simulink model "Kinect_Block_modified"  (R2012b)
settings: Solver=ode45  StartTime=0.0  StopTime=inf  RelTol=1e-3
undefined symbols (not defined in the file or in its folder): gray
libraries: nid_lib x2, visionsinks x1, utility x1
settings Model: Creator=Eka  LastModifiedBy=Eka

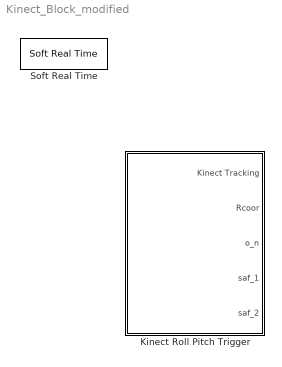
== system Kinect_Block_modified ==
  Kinect Roll Pitch Trigger : Subsystem
  Soft Real Time : utility/Soft Real Time  x=0.8

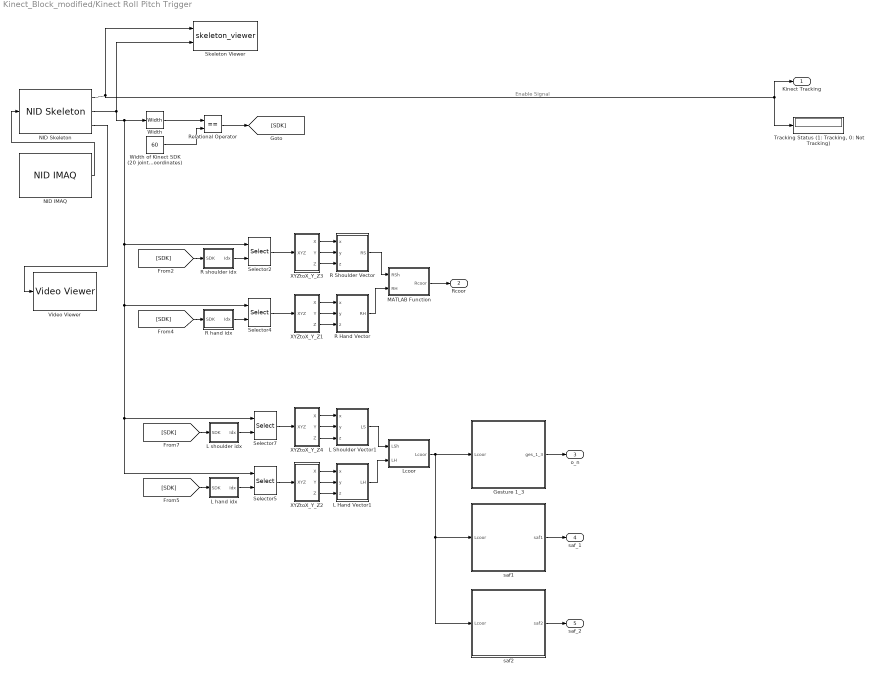
== system Kinect_Block_modified/Kinect Roll Pitch Trigger ==
  note: Enable Signal
  Gesture 1_3 : MATLAB Function  TreatAsAtomicUnit=on
  L Hand Vector1 : MATLAB Function  TreatAsAtomicUnit=on
  L Shoulder Vector1 : MATLAB Function  TreatAsAtomicUnit=on
  L hand idx : Subsystem
  L shoulder idx : Subsystem
  Lcoor : MATLAB Function  TreatAsAtomicUnit=on
  MATLAB Function : MATLAB Function  TreatAsAtomicUnit=on
  NID IMAQ : nid_lib/NID IMAQ  imaq_depth=off  imaq_motion=off  imaq_image=off  view_point=off  imaq_skeleton=on  imaq_ir=off  mirror_image=off  imaq_sample_time=1/25  res_fps=VGA (640x480): 30 FPS  needPsiPose=off  angle_input=off  angle=0  angle_read=off  near_mode=on  seated_mode=on  skeleton_smooth=[1.0 0.5 0.5 0.05 0.04]  infer_skeleton=on
  NID Skeleton : nid_lib/NID Skeleton  num_of_skeleton_tracking=1  conv_XYZ_RW=on  viewer=on
  R Hand Vector : MATLAB Function  TreatAsAtomicUnit=on
  R Shoulder Vector : MATLAB Function  TreatAsAtomicUnit=on
  R hand idx : Subsystem
  R shoulder idx : Subsystem
  Relational Operator : RelationalOperator  Operator===  OutDataTypeStr=boolean
  Selector{2,4..5,7} (4 alike) : Selector  NumberOfDimensions=3  InputPortWidth=3  IndexOptions=Select all,Index vector (port),Select all  Indices=[1 3],1,1  OutputSizes=1,1,1
  Skeleton Viewer : M-S-Function  FunctionName=skeleton_viewer
      mask Display:
      | disp('Skeleton\nViewer')
      | 
      | port_label('input', 1, 'Tracking')
      | port_label('input', 2, 'Skeleton')
  "Tracking Status (1: Tracking, 0: Not Tracking)" : Display
  Video Viewer : visionsinks/Video Viewer  inputType=Obsolete7b  imagePorts=One multidimensional signal  useColorMap=off  colormapValue=gray(256)  specRange=off  minInputVal=0  maxInputVal=255  FigPos=[578 777 794 668]  AxisZoom=on  trueSizedOnce=off  OpenAtMdlStart=on  DefaultConfigurationName=vipscopes.VideoViewerScopeCfg
  Width : Width
  Width of Kinect SDK (20 joints x 3 coordinates) : Constant  Value=60
  XYZtoX_Y_Z1 : Subsystem
  XYZtoX_Y_Z2 : Subsystem
  XYZtoX_Y_Z3 : Subsystem
  XYZtoX_Y_Z4 : Subsystem
  saf1 : MATLAB Function  TreatAsAtomicUnit=on
  saf2 : MATLAB Function  TreatAsAtomicUnit=on
  Kinect Tracking : Outport
  Rcoor : Outport  Port=2
  o_n : Outport  Port=3
  saf_1 : Outport  Port=4
  saf_2 : Outport  Port=5
  wires:
  [SDK] -> R hand idx/1(SDK)
  R hand idx/1(Idx) -> Selector4/2
  [SDK] -> R shoulder idx/1(SDK)
  R shoulder idx/1(Idx) -> Selector2/2
  NID Skeleton/1 -> "Tracking Status (1: Tracking, 0: Not Tracking)"/1, Kinect Tracking/1, Skeleton Viewer/1
  Relational Operator/1 -> [SDK]
  Width of Kinect SDK (20 joints x 3 coordinates)/1 -> Relational Operator/2
  Width/1 -> Relational Operator/1
  NID IMAQ/1 -> NID Skeleton/1
  [SDK] -> L hand idx/1(SDK)
  [SDK] -> L shoulder idx/1(SDK)
  L hand idx/1(Idx) -> Selector5/2
  L shoulder idx/1(Idx) -> Selector7/2
  NID Skeleton/3 -> Video Viewer/1
  NID Skeleton/2 -> Selector5/1, Selector7/1, Selector4/1, Selector2/1, Width/1, Skeleton Viewer/2
  MATLAB Function/1(Rcoor) -> Rcoor/1
  Selector2/1 -> XYZtoX_Y_Z3/1(XYZ)
  Selector4/1 -> XYZtoX_Y_Z1/1(XYZ)
  XYZtoX_Y_Z1/1(X) -> R Hand Vector/1(x)
  XYZtoX_Y_Z1/2(Y) -> R Hand Vector/2(y)
  XYZtoX_Y_Z1/3(Z) -> R Hand Vector/3(z)
  XYZtoX_Y_Z3/3(Z) -> R Shoulder Vector/3(z)
  XYZtoX_Y_Z3/2(Y) -> R Shoulder Vector/2(y)
  XYZtoX_Y_Z3/1(X) -> R Shoulder Vector/1(x)
  R Shoulder Vector/1(RS) -> MATLAB Function/1(RSh)
  R Hand Vector/1(RH) -> MATLAB Function/2(RH)
  XYZtoX_Y_Z2/1(X) -> L Hand Vector1/1(x)
  XYZtoX_Y_Z2/2(Y) -> L Hand Vector1/2(y)
  XYZtoX_Y_Z2/3(Z) -> L Hand Vector1/3(z)
  XYZtoX_Y_Z4/3(Z) -> L Shoulder Vector1/3(z)
  XYZtoX_Y_Z4/2(Y) -> L Shoulder Vector1/2(y)
  XYZtoX_Y_Z4/1(X) -> L Shoulder Vector1/1(x)
  Selector7/1 -> XYZtoX_Y_Z4/1(XYZ)
  Selector5/1 -> XYZtoX_Y_Z2/1(XYZ)
  L Shoulder Vector1/1(LS) -> Lcoor/1(LSh)
  L Hand Vector1/1(LH) -> Lcoor/2(LH)
  Lcoor/1(Lcoor) -> Gesture 1_3/1(Lcoor), saf2/1(Lcoor), saf1/1(Lcoor)
  saf1/1(saf1) -> saf_1/1
  saf2/1(saf2) -> saf_2/1
  Gesture 1_3/1(ges_1_3) -> o_n/1

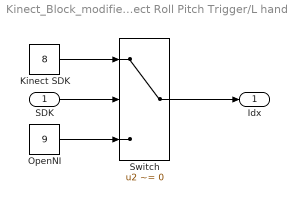
== system Kinect_Block_modified/Kinect Roll Pitch Trigger/L hand idx ==
  SDK : Inport
  Kinect SDK : Constant  Value=8
  OpenNI : Constant  Value=9
  Switch : Switch  Criteria=u2 ~= 0
  Idx : Outport
  wires:
  Kinect SDK/1 -> Switch/1
  OpenNI/1 -> Switch/3
  SDK/1 -> Switch/2
  Switch/1 -> Idx/1

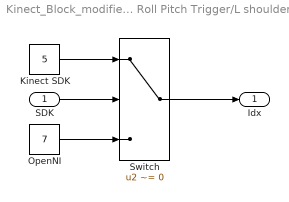
== system Kinect_Block_modified/Kinect Roll Pitch Trigger/L shoulder idx ==
  SDK : Inport
  Kinect SDK : Constant  Value=5
  OpenNI : Constant  Value=7
  Switch : Switch  Criteria=u2 ~= 0
  Idx : Outport
  wires:
  Kinect SDK/1 -> Switch/1
  OpenNI/1 -> Switch/3
  SDK/1 -> Switch/2
  Switch/1 -> Idx/1

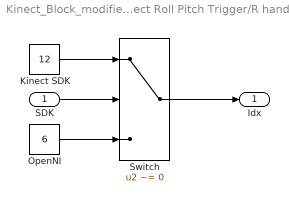
== system Kinect_Block_modified/Kinect Roll Pitch Trigger/R hand idx ==
  SDK : Inport
  Kinect SDK : Constant  Value=12
  OpenNI : Constant  Value=6
  Switch : Switch  Criteria=u2 ~= 0
  Idx : Outport
  wires:
  Switch/1 -> Idx/1
  SDK/1 -> Switch/2
  OpenNI/1 -> Switch/3
  Kinect SDK/1 -> Switch/1

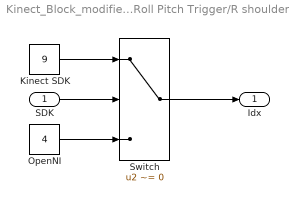
== system Kinect_Block_modified/Kinect Roll Pitch Trigger/R shoulder idx ==
  SDK : Inport
  Kinect SDK : Constant  Value=9
  OpenNI : Constant  Value=4
  Switch : Switch  Criteria=u2 ~= 0
  Idx : Outport
  wires:
  Switch/1 -> Idx/1
  SDK/1 -> Switch/2
  OpenNI/1 -> Switch/3
  Kinect SDK/1 -> Switch/1

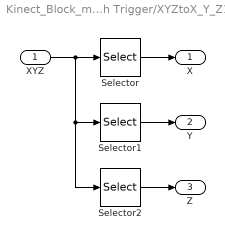
== system Kinect_Block_modified/Kinect Roll Pitch Trigger/XYZtoX_Y_Z1 ==
  XYZ : Inport
  Selector : Selector  NumberOfDimensions=3  InputPortWidth=3  IndexOptions=Index vector (dialog),Index vector (dialog),Index vector (dialog)  Indices=1,1,1  OutputSizes=1,1,1
  Selector1 : Selector  NumberOfDimensions=3  InputPortWidth=3  IndexOptions=Index vector (dialog),Index vector (dialog),Index vector (dialog)  Indices=1,1,2  OutputSizes=1,1,1
  Selector2 : Selector  NumberOfDimensions=3  InputPortWidth=3  IndexOptions=Index vector (dialog),Index vector (dialog),Index vector (dialog)  Indices=1,1,3  OutputSizes=1,1,1
  X : Outport
  Y : Outport  Port=2
  Z : Outport  Port=3
  wires:
  Selector2/1 -> Z/1
  Selector1/1 -> Y/1
  Selector/1 -> X/1
  XYZ/1 -> Selector2/1, Selector1/1, Selector/1

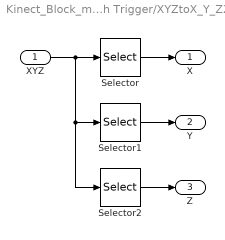
== system Kinect_Block_modified/Kinect Roll Pitch Trigger/XYZtoX_Y_Z2 ==
  XYZ : Inport
  Selector : Selector  NumberOfDimensions=3  InputPortWidth=3  IndexOptions=Index vector (dialog),Index vector (dialog),Index vector (dialog)  Indices=1,1,1  OutputSizes=1,1,1
  Selector1 : Selector  NumberOfDimensions=3  InputPortWidth=3  IndexOptions=Index vector (dialog),Index vector (dialog),Index vector (dialog)  Indices=1,1,2  OutputSizes=1,1,1
  Selector2 : Selector  NumberOfDimensions=3  InputPortWidth=3  IndexOptions=Index vector (dialog),Index vector (dialog),Index vector (dialog)  Indices=1,1,3  OutputSizes=1,1,1
  X : Outport
  Y : Outport  Port=2
  Z : Outport  Port=3
  wires:
  XYZ/1 -> Selector/1, Selector1/1, Selector2/1
  Selector/1 -> X/1
  Selector1/1 -> Y/1
  Selector2/1 -> Z/1

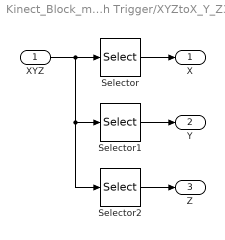
== system Kinect_Block_modified/Kinect Roll Pitch Trigger/XYZtoX_Y_Z3 ==
  XYZ : Inport
  Selector : Selector  NumberOfDimensions=3  InputPortWidth=3  IndexOptions=Index vector (dialog),Index vector (dialog),Index vector (dialog)  Indices=1,1,1  OutputSizes=1,1,1
  Selector1 : Selector  NumberOfDimensions=3  InputPortWidth=3  IndexOptions=Index vector (dialog),Index vector (dialog),Index vector (dialog)  Indices=1,1,2  OutputSizes=1,1,1
  Selector2 : Selector  NumberOfDimensions=3  InputPortWidth=3  IndexOptions=Index vector (dialog),Index vector (dialog),Index vector (dialog)  Indices=1,1,3  OutputSizes=1,1,1
  X : Outport
  Y : Outport  Port=2
  Z : Outport  Port=3
  wires:
  XYZ/1 -> Selector/1, Selector1/1, Selector2/1
  Selector/1 -> X/1
  Selector1/1 -> Y/1
  Selector2/1 -> Z/1

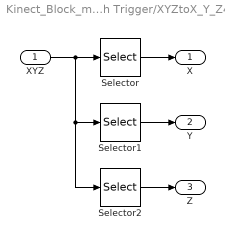
== system Kinect_Block_modified/Kinect Roll Pitch Trigger/XYZtoX_Y_Z4 ==
  XYZ : Inport
  Selector : Selector  NumberOfDimensions=3  InputPortWidth=3  IndexOptions=Index vector (dialog),Index vector (dialog),Index vector (dialog)  Indices=1,1,1  OutputSizes=1,1,1
  Selector1 : Selector  NumberOfDimensions=3  InputPortWidth=3  IndexOptions=Index vector (dialog),Index vector (dialog),Index vector (dialog)  Indices=1,1,2  OutputSizes=1,1,1
  Selector2 : Selector  NumberOfDimensions=3  InputPortWidth=3  IndexOptions=Index vector (dialog),Index vector (dialog),Index vector (dialog)  Indices=1,1,3  OutputSizes=1,1,1
  X : Outport
  Y : Outport  Port=2
  Z : Outport  Port=3
  wires:
  Selector2/1 -> Z/1
  Selector1/1 -> Y/1
  Selector/1 -> X/1
  XYZ/1 -> Selector2/1, Selector1/1, Selector/1

== matlab function Kinect_Block_modified/Kinect Roll Pitch Trigger/L Hand Vector1 ==
  data: x input; y input; z input; LH output
function LH = fcn(x,y,z)
LH = [x,y,z];

== matlab function Kinect_Block_modified/Kinect Roll Pitch Trigger/Lcoor ==
  data: LSh input; LH input; Lcoor output
function Lcoor = fcn(LSh, LH)
%#codegen

Lcoor = (LH - LSh)*10;

== matlab function Kinect_Block_modified/Kinect Roll Pitch Trigger/MATLAB Function ==
  data: RSh input; RH input; Rcoor output
function Rcoor = fcn(RSh, RH)

x_axis = (RH(1) - RSh(1))*(-5);
y_axis = ((RH(3) - RSh(3))+4)*4/3;
z_axis = (((RH(2) - RSh(2))+1)*1.8/7)-1.5;
Rcoor = [x_axis, y_axis, z_axis];

== matlab function Kinect_Block_modified/Kinect Roll Pitch Trigger/L Shoulder Vector1 ==
  data: x input; y input; z input; LS output
function LS = fcn(x,y,z)
LS = [x,y,z];

== matlab function Kinect_Block_modified/Kinect Roll Pitch Trigger/R Shoulder Vector ==
  data: x input; y input; z input; RS output
function RS = fcn(x,y,z)
RS = [x,y,z];

== matlab function Kinect_Block_modified/Kinect Roll Pitch Trigger/R Hand Vector ==
  data: x input; y input; z input; RH output
function RH = fcn(x,y,z)
RH = [x,y,z];

== matlab function Kinect_Block_modified/Kinect Roll Pitch Trigger/Gesture 1_3 ==
  data: Lcoor input; ges_1_3 output
function ges_1_3 = fcn(Lcoor)
%#codegen

if (Lcoor(1) > 0 & Lcoor(1) < 2.5 & ...
    Lcoor(2) > -1 & Lcoor(2) < 1 & ...
    Lcoor(3) > -4.5 & Lcoor(3) < 0)
    
    ges_1_3 = 1;

else
    
    ges_1_3 = 0;

end

== matlab function Kinect_Block_modified/Kinect Roll Pitch Trigger/saf1 ==
  data: Lcoor input; saf1 output
function saf1 = fcn(Lcoor)
%#codegen

if (Lcoor(1) > 4.5)
    
    saf1 = 1;

else
    
    saf1 = 0;

end

== matlab function Kinect_Block_modified/Kinect Roll Pitch Trigger/saf2 ==
  data: Lcoor input; saf2 output
function saf2 = fcn(Lcoor)
%#codegen

if (Lcoor(2) > 1.5)
    
    saf2 = 1;

else
    
    saf2 = 0;

end
